simulink model "fuzzypd9"  (R2018a)
settings: Solver=VariableStepAuto  StartTime=0.0  StopTime=10.0  RelTol=1e-3
undefined symbols (not defined in the file or in its folder): kd0_T, kp0_T
libraries: simulink x1
settings Model: Creator=wangkingsheng  LastModifiedBy=wangkingsheng

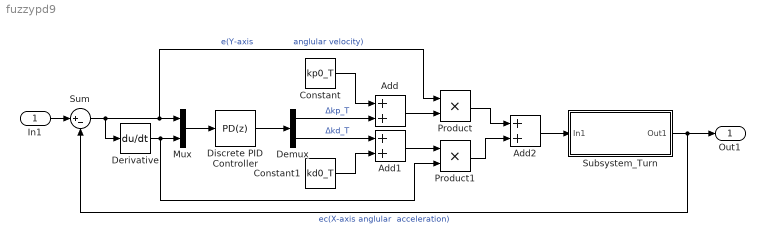
== system fuzzypd9 ==
  In1 : Inport
  Add : Sum
  Add1 : Sum
  Add2 : Sum
  Constant : Constant  Value=kp0_T
  Constant1 : Constant  Value=kd0_T
  Demux : Demux  Outputs=2
  Derivative : Derivative
  Discrete PID Controller : simulink/Continuous/PID Controller  Controller=PD  TimeDomain=Discrete-time  SampleTime=-1  IntegratorMethod=Forward Euler  FilterMethod=Forward Euler  Form=Parallel  UseFilter=on  ControllerParametersSource=internal  P=1  I=1  D=0  N=100  InitialConditionSource=internal  InitialConditionForIntegrator=0  InitialConditionForFilter=0  ExternalReset=none  LimitOutput=off  UpperSaturationLimit=inf  LowerSaturationLimit=-inf  LinearizeAsGain=off  AntiWindupMode=none  Kb=1  TrackingMode=off  Kt=1  PParamMin=[]  PParamMax=[]  IParamMin=[]  IParamMax=[]  DParamMin=[]  DParamMax=[]  NParamMin=[]  NParamMax=[]  KbParamMin=[]  KbParamMax=[]  KtParamMin=[]  KtParamMax=[]  POutMin=[]  POutMax=[]  IOutMin=[]  IOutMax=[]  DOutMin=[]  DOutMax=[]  NOutMin=[]  NOutMax=[]  KbOutMin=[]  KbOutMax=[]  KtOutMin=[]  KtOutMax=[]  IntegratorOutMin=[]  IntegratorOutMax=[]  FilterOutMin=[]  FilterOutMax=[]  SumOutMin=[]  SumOutMax=[]  SumI1OutMin=[]  SumI1OutMax=[]  SumI2OutMin=[]  SumI2OutMax=[]  SumI3OutMin=[]  SumI3OutMax=[]  SumDOutMin=[]  SumDOutMax=[]  SaturationOutMin=[]  SaturationOutMax=[]  IntegratorContinuousStateAttributes=''  IntegratorStateMustResolveToSignalObject=off  IntegratorRTWStateStorageClass=Auto  FilterContinuousStateAttributes=''  FilterStateMustResolveToSignalObject=off  FilterRTWStateStorageClass=Auto  DifferentiatorICPrevScaledInput=0  DifferentiatorOutMin=[]  DifferentiatorOutMax=[]  FilterDiffOutCoefMin=[]  FilterDiffOutCoefMax=[]  SumDenOutMin=[]  SumDenOutMax=[]  SumNumOutMin=[]  SumNumOutMax=[]  ReciprocalOutMin=[]  ReciprocalOutMax=[]  DivideOutMin=[]  DivideOutMax=[]  TunerSelectOption=Transfer Function Based (PID Tuner App)
  Mux : Mux  Inputs=2
  Product : Product
  Product1 : Product
  Subsystem_Turn : Subsystem
  Sum : Sum  Inputs=|+-
  Out1 : Outport
  wires:
  In1/1 -> Sum/1
  Discrete PID Controller/1 -> Demux/1
  Mux/1 -> Discrete PID Controller/1
  Demux/1 -> Add/2  "Δkp_T"
  Demux/2 -> Add1/1  "Δkd_T"
  Constant/1 -> Add/1
  Constant1/1 -> Add1/2
  Add2/1 -> Subsystem_Turn/1(In1)
  Add/1 -> Product/2
  Add1/1 -> Product1/1
  Product1/1 -> Add2/2
  Product/1 -> Add2/1
  Subsystem_Turn/1(Out1) -> Out1/1, Sum/2  "ec(X-axis anglular  acceleration)"
  Sum/1 -> Derivative/1, Product/1, Mux/1  "e(Y-axis               anglular velocity)"
  Derivative/1 -> Product1/2, Mux/2

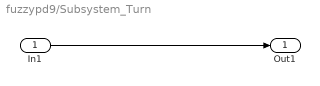
== system fuzzypd9/Subsystem_Turn ==
  In1 : Inport
  Out1 : Outport
  wires:
  In1/1 -> Out1/1
